simulink library "NoiseLib_2019"  (R2016a)
settings: Solver=ode45  StartTime=0.0  StopTime=10.0  RelTol=1e-3
undefined symbols (not defined in the file): dt, htp, Tsk
libraries: dspsrcs4 x5
settings Model: Creator=Bornitz  LastModifiedBy=Bornitz
settings DataIOCC: LimitDataPoints=on
settings DebuggingCC: AllowSymbolicDim=off

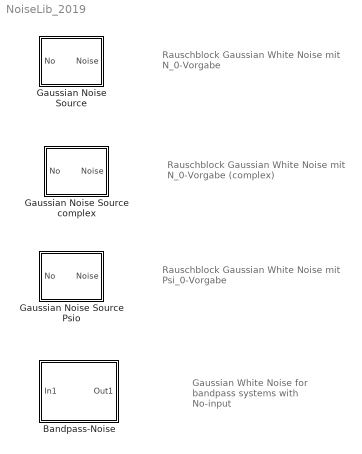
== system NoiseLib_2019 ==
  note: Rauschblock Gaussian White Noise
      |  mit Psi_0-Vorgabe
  note: Rauschblock Gaussian White Noise
      |  mit N_0-Vorgabe
  note: Rauschblock Gaussian White Noise
      |  mit N_0-Vorgabe (complex)
  note: Gaussian White Noise
      |  for bandpass systems
      |  with No-input
  Bandpass-Noise : Subsystem
      mask help: Der Block erzeugt Gaussverteiltes Weisses Rauschen um die Trägerfrequenz f0 mit der Bandbreite 2xW.
      mask Help:
      | Im Workspace zu definieren sind:
      | f0 als Trägerfrequenz,
      | W als halbe Bandbreite,
      | fs1 als Abtastfrequenz im hochgemischten Bereich
      | dt= 1/fs1 als TimeStep der Simulation
      mask Display:
      | plot(0,0,100,100,[95 5 10 10 10 (100-15)*[0:1/30:1]+10],[75 75 75 70 95 70    58 76 77 63 86 86 74 78 76 73 82 69 96 73 76 85 75 74 66 77 61 82 91 68    83 87 59 60 80 71]);
      | disp('\n\n Gaussian Noise\n defined\n frequency range')
  Gaussian Noise Source : Subsystem
      mask Display:
      | plot(0,0,100,100,[95 5 10 10 10 (100-15)*[0:1/30:1]+10],[75 75 75 70 95 70    58 76 77 63 86 86 74 78 76 73 82 69 96 73 76 85 75 74 66 77 61 82 91 68    83 87 59 60 80 71]);
      | disp('\n\nGaussian')
      | port_label('input',1,'No')
      | port_label('output',1,'noise')
  Gaussian Noise Source Psio : Subsystem
      mask Display:
      | plot(0,0,100,100,[95 5 10 10 10 (100-15)*[0:1/30:1]+10],[75 75 75 70 95 70    58 76 77 63 86 86 74 78 76 73 82 69 96 73 76 85 75 74 66 77 61 82 91 68    83 87 59 60 80 71]);
      | disp('\n\nGaussian')
      | port_label('input',1,'Psio')
      | port_label('output',1,'noise')
  Gaussian Noise Source complex : Subsystem
      mask Display:
      | plot(0,0,100,100,[95 5 10 10 10 (100-15)*[0:1/30:1]+10],[75 75 75 70 95 70    58 76 77 63 86 86 74 78 76 73 82 69 96 73 76 85 75 74 66 77 61 82 91 68    83 87 59 60 80 71]);
      | disp('\n\nGaussian')
      | port_label('input',1,'No')
      | port_label('output',1,'noise')

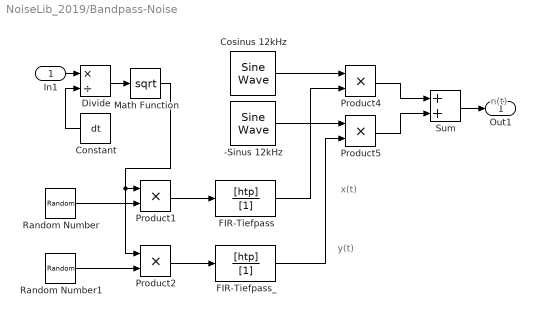
== system NoiseLib_2019/Bandpass-Noise ==
  note: n(t)
  note: x(t)
  note: y(t)
  In1 : Inport
  -Sinus 12kHz : dspsrcs4/Sine Wave  Amplitude=-1  Frequency=12000  Phase=0  SampleMode=Discrete  OutComplex=Real  CompMethod=Trigonometric fcn  TableSize=Speed  SampleTime=Tsk  SamplesPerFrame=1  ResetState=Restart at time zero  OutputFrames=on  dataType=double  wordLen=16  udDataType=sfix(16)  fracBitsMode=Best precision  numFracBits=15  OutDataTypeStr=double  LastOutDataTypeStr=double
  Constant : Constant  Value=dt
  Cosinus 12kHz : dspsrcs4/Sine Wave  Amplitude=1  Frequency=12000  Phase=pi/2  SampleMode=Discrete  OutComplex=Real  CompMethod=Trigonometric fcn  TableSize=Speed  SampleTime=Tsk  SamplesPerFrame=1  ResetState=Restart at time zero  OutputFrames=on  dataType=double  wordLen=16  udDataType=sfix(16)  fracBitsMode=Best precision  numFracBits=15  OutDataTypeStr=double  LastOutDataTypeStr=double
  Divide : Product  Inputs=*/
  FIR-Tiefpass : DiscreteFilter  Numerator=[htp]  Denominator=[1]  SampleTime=Tsk
  FIR-Tiefpass_ : DiscreteFilter  Numerator=[htp]  Denominator=[1]  SampleTime=Tsk
  Math Function : Math  Operator=sqrt  SaturateOnIntegerOverflow=on
  Product{1..2,4..5} (4 alike) : Product  SaturateOnIntegerOverflow=on  RndMeth=Zero  InputSameDT=on  OutDataTypeStr=Inherit: Same as first input
  Random Number : RandomNumber  Seed=136783  SampleTime=Tsk
  Random Number1 : RandomNumber  Seed=915638  SampleTime=Tsk
  Sum : Sum  SaturateOnIntegerOverflow=on  InputSameDT=on  OutDataTypeStr=Inherit: Same as first input
  Out1 : Outport
  wires:
  Product5/1 -> Sum/2
  Product4/1 -> Sum/1
  FIR-Tiefpass/1 -> Product4/2
  FIR-Tiefpass_/1 -> Product5/2
  Product1/1 -> FIR-Tiefpass/1
  Product2/1 -> FIR-Tiefpass_/1
  -Sinus 12kHz/1 -> Product5/1
  Cosinus 12kHz/1 -> Product4/1
  Sum/1 -> Out1/1
  In1/1 -> Divide/1
  Random Number/1 -> Product1/2
  Random Number1/1 -> Product2/2
  Divide/1 -> Math Function/1
  Constant/1 -> Divide/2
  Math Function/1 -> Product1/1, Product2/1

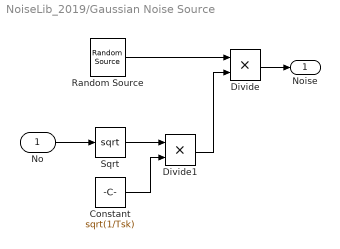
== system NoiseLib_2019/Gaussian Noise Source ==
  No : Inport
  Constant : Constant  Value=sqrt(1/Tsk)
  Divide : Product  Inputs=**
  Divide1 : Product  Inputs=**
  Random Source : dspsrcs4/Random Source  SrcType=Gaussian  NormMethod=Ziggurat  CltLength=12  MinVal=0  MaxVal=1  MeanVal=0  VarVal=1  RepMode=Specify seed  rawSeed=31  IsInherit=off  SampMode=Discrete  SampTime=Tsk  SampFrame=1  DataType=Double  OutComplex=Real  OutputFrames=off
  Sqrt : Sqrt  SaturateOnIntegerOverflow=on
  Noise : Outport
  wires:
  Random Source/1 -> Divide/1
  Divide/1 -> Noise/1
  Divide1/1 -> Divide/2
  Constant/1 -> Divide1/2
  Sqrt/1 -> Divide1/1
  No/1 -> Sqrt/1

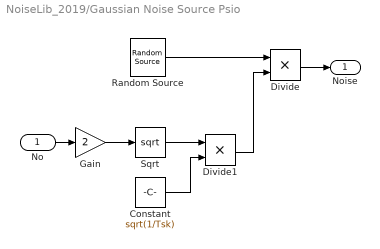
== system NoiseLib_2019/Gaussian Noise Source Psio ==
  No : Inport
  Constant : Constant  Value=sqrt(1/Tsk)
  Divide : Product  Inputs=**
  Divide1 : Product  Inputs=**
  Gain : Gain  Gain=2
  Random Source : dspsrcs4/Random Source  SrcType=Gaussian  NormMethod=Ziggurat  CltLength=12  MinVal=0  MaxVal=1  MeanVal=0  VarVal=1  RepMode=Not repeatable  rawSeed=1  IsInherit=off  SampMode=Discrete  SampTime=Tsk  SampFrame=1  DataType=Double  OutComplex=Real  OutputFrames=off
  Sqrt : Sqrt  SaturateOnIntegerOverflow=on
  Noise : Outport
  wires:
  No/1 -> Gain/1
  Sqrt/1 -> Divide1/1
  Constant/1 -> Divide1/2
  Divide1/1 -> Divide/2
  Divide/1 -> Noise/1
  Random Source/1 -> Divide/1
  Gain/1 -> Sqrt/1

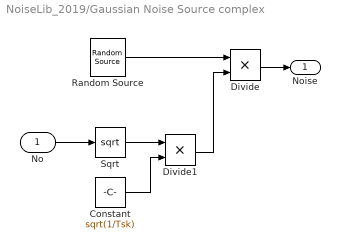
== system NoiseLib_2019/Gaussian Noise Source complex ==
  No : Inport
  Constant : Constant  Value=sqrt(1/Tsk)
  Divide : Product  Inputs=**
  Divide1 : Product  Inputs=**
  Random Source : dspsrcs4/Random Source  SrcType=Gaussian  NormMethod=Ziggurat  CltLength=12  MinVal=0  MaxVal=1  MeanVal=0  VarVal=1  RepMode=Not repeatable  rawSeed=1  IsInherit=off  SampMode=Discrete  SampTime=Tsk  SampFrame=1  DataType=Double  OutComplex=Complex  OutputFrames=off
  Sqrt : Sqrt  SaturateOnIntegerOverflow=on
  Noise : Outport
  wires:
  Random Source/1 -> Divide/1
  Divide/1 -> Noise/1
  Divide1/1 -> Divide/2
  Constant/1 -> Divide1/2
  Sqrt/1 -> Divide1/1
  No/1 -> Sqrt/1
